simulink model "randament_pompa"  (R2022b)
settings: Solver=VariableStepAuto  StartTime=0.0  StopTime=10.0  RelTol=1e-3
values from neighbouring files (symbols this model uses):
  keta = 8*10^(-5)    (= 8e-05)    [run_first.m]
settings Model: Creator=fabian  LastModifiedBy=fabian

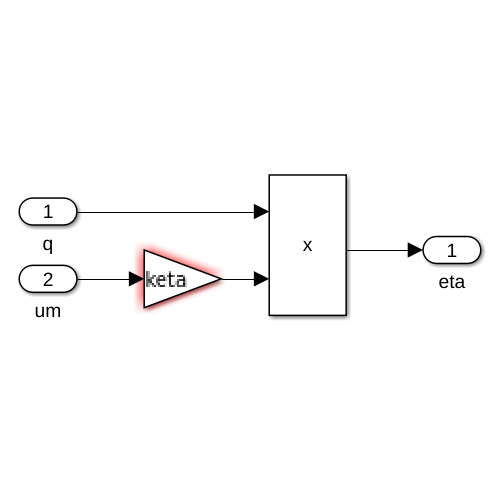
[thumbnail: Simulink's stored preview of the top-level diagram]
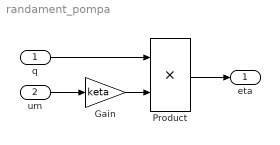
== system randament_pompa ==
  q : Inport
  um : Inport  Port=2
  Gain : Gain  Gain=keta
  Product : Product
  eta : Outport
  wires:
  Product/1 -> eta/1
  Gain/1 -> Product/2
  um/1 -> Gain/1
  q/1 -> Product/1
